simulink model "ploop_test"  (Simulink 7.9)
settings: Solver=ode15s  StartTime=0.0  StopTime=1  RelTol=1e-3
undefined symbols (not defined in the file or in its folder): G
libraries: roblocks x1
settings Model: Creator=pic  LastModifiedBy=corkep
settings DataIOCC: LimitDataPoints=off  OutputOption=SpecifiedOutputTimes  OutputTimes=[0:0.001:1]'
settings DebuggingCC: FcnCallInpInsideContextMsg=Use local settings  StrictBusMsg=Warning
settings GRTTargetCC: CombineOutputUpdateFcns=off  GRTInterface=on

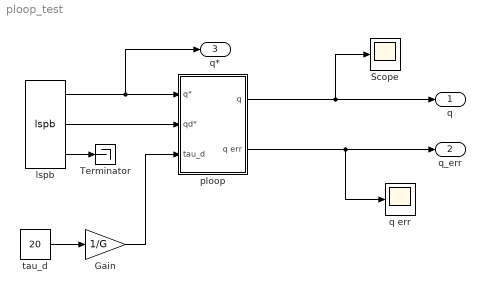
== system ploop_test ==
  Gain : Gain  Gain=1/G
  Scope : Scope
      settings: YMin=0  YMax=55
  Terminator : Terminator
  lspb : roblocks/Trajectory/lspb  q0=0  qf=0.5*G  tmax=1
  ploop : Subsystem
  q err : Scope
      settings: TimeRange=1  YMin=-0.5  YMax=8
  tau_d : Constant  Value=20
  q : Outport
  q_err : Outport  Port=2
  q* : Outport  Port=3
  wires:
  ploop/1(q) -> q/1, Scope/1
  ploop/2(q err) -> q_err/1, q err/1
  tau_d/1 -> Gain/1
  lspb/1 -> q*/1, ploop/1(q*)
  Gain/1 -> ploop/3(tau_d)
  lspb/3 -> Terminator/1
  lspb/2 -> ploop/2(qd*)

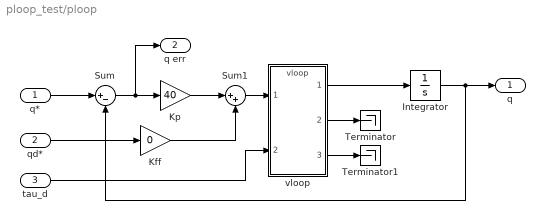
== system ploop_test/ploop ==
  q* : Inport
  qd* : Inport  Port=2
  tau_d : Inport  Port=3
  Integrator : Integrator
  Kff : Gain  Gain=0
  Kp : Gain  Gain=40
  Sum : Sum  Inputs=|+-
  Sum1 : Sum  Inputs=|++
  Terminator : Terminator
  Terminator1 : Terminator
  vloop : ModelReference  ModelNameDialog=vloop  ModelReferenceVersion=1.8  CopyOfModelName=vloop  DefaultDataLogging=off
  q : Outport
  q err : Outport  Port=2
  wires:
  tau_d/1 -> vloop/2
  Sum/1 -> Kp/1, q err/1
  vloop/1 -> Integrator/1
  Integrator/1 -> q/1, Sum/2
  q*/1 -> Sum/1
  vloop/2 -> Terminator/1
  vloop/3 -> Terminator1/1
  Kp/1 -> Sum1/1
  Sum1/1 -> vloop/1
  qd*/1 -> Kff/1
  Kff/1 -> Sum1/2
